simulink model "automatic_transmission_control"  (R2020b)
settings: Solver=ode5  StartTime=0.0  StopTime=30  FixedStep=0.001  RelTol=1e-3
PreLoadFcn:
  | initialization
values from neighbouring files (symbols this model uses):
  CONVERTER_DATA = [0 137.4652089938063 2.2319999999999998;0.1 137.06501915685197 2.075;0.2 135.86444964598905 1.975;0.30000000000000004 135.66435472751189 1.8459999999999999;0.4 137.56525645304487 1.72;0.5 140.36658531172509 1.564;0.60000000000000009 145.26891081441539 1.409;0.70000000000000007 152.87251771654735 1.254;0.8 162.97731109964374 1.0959999999999999;0.81 164.2779280697452 1.08;0.82000000000000006 166.178 ...(+346 chars)    [initialization.m]
  DOWN_TABLE = [0 5 20 35;0 5 20 35;0 5 25 40;0 5 30 50;0 30 50 80;0 30 50 80]    [initialization.m]
  DOWN_TH_BP = [0;5;40;50;90;100]    [initialization.m]
  EMAP = [-40 -44 -49 -53 -57 -61 -65 -70 -74 -78 -82;215 117 85 66 44 29 10 -2 -13 -22 -32;245 208 178 148 122 104 85 66 48 33 18;264 260 241 219 193 167 152 133 119 96 85;264 279 282 275 260 238 223 208 189 171 152;267 290 293 297 290 275 260 256 234 212 193;267 297 305 305 305 301 293 282 267 249 226;267 301 308 312 319 323 319 316 297 279 253;267 301 312 319 327 327 327 327 312 293 267;267 301 312 319  ...(+28 chars)    [initialization.m]
  Iei = 0.021991488283555904    (= 0.0219914882836)    [initialization.m]
  NE_VEC = [799.99999999999989 1200 1599.9999999999998 1999.9999999999998 2400 2800.0000000000005 3199.9999999999995 3599.9999999999995 3999.9999999999995 4400 4800]    [initialization.m]
  TH_VEC = [0;20;30;40;50;60;70;80;90;100]    [initialization.m]
  UP_TABLE = [10 30 50 1.0E+6;10 30 50 1.0E+6;15 30 50 1.0E+6;23 41 60 1.0E+6;40 70 100 1.0E+6;40 70 100 1.0E+6]    [initialization.m]
  UP_TH_BP = [0;25;35;50;90;100]    [initialization.m]
  VEHICLE_DATA = [3.23;40;0.02;1;12.094147857312473;0]    [initialization.m]
undefined symbols (not defined in the file or in its folder): sigbuilder_block
settings Model: Creator=Vrunda M Balgi  LastModifiedBy=Vrunda M Balgi

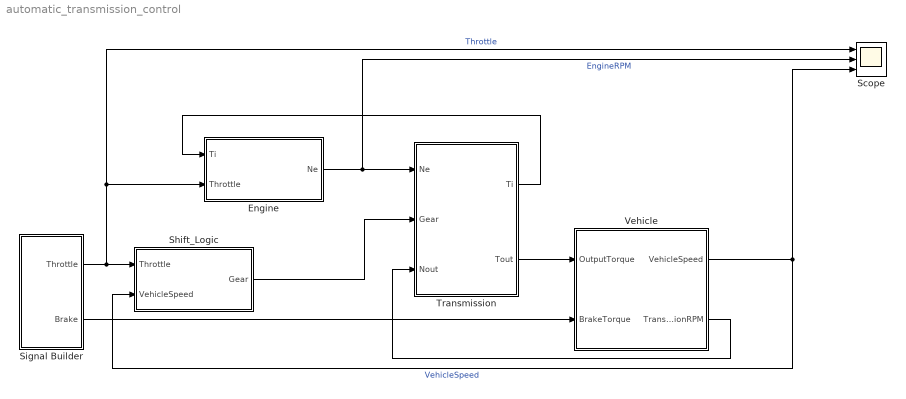
== system automatic_transmission_control ==
  Engine : Subsystem
  Scope : Scope  NumInputPorts=3
  Shift_Logic : Stateflow chart  TreatAsAtomicUnit=on
  Signal Builder : Subsystem  Tag=STV Subsys  LoadFcn=sigbuilder_block('load',[574.2 159.6 550.8 400.2 ]);  StartFcn=sigbuilder_block('start');  StopFcn=sigbuilder_block('stop');  ClipboardFcn=sigbuilder_block('clipboard');  mask(Sigbuilder block){tuvar=[0:10]}
      mask help: Simulink:masks:SigbuilderBlock_MD
      mask init:
      | if ~strcmp(get_param(bdroot(gcbh),'SimulationStatus'),'stopped') tuvar = sigbuilder_block('maskInit'); end
      settings: CopyFcn=sigbuilder_block('copy');  DeleteFcn=sigbuilder_block('delete');  ModelCloseFcn=sigbuilder_block('modelClose');  PreSaveFcn=sigbuilder_block('preSave');  PauseFcn=sigbuilder_block('pause');  ContinueFcn=sigbuilder_block('continue');  NameChangeFcn=sigbuilder_block('namechange');  OpenFcn=sigbuilder_block('open',[574.2 159.6 550.8 400.2 ]);  CloseFcn=sigbuilder_block('close');
      mask Display: plot(0, 0, 100, 100,[2, 2, 32, 32, 2], [68, 8, 8, 68, 68],[32, 2], [38, 38], [32, 19, 2],[53, 60, 44], [32, 17, 17, 2],[16, 16, 31, 31]);txt = getActiveGroup(gcbh);text(2, 100, txt,'verticalAlignment', 'top');
  Transmission : Subsystem
  Vehicle : Subsystem
  wires:
  Transmission/1(Ti) -> Engine/1(Ti)
  Signal Builder/1(Throttle) -> Scope/1, Engine/2(Throttle), Shift_Logic/1(Throttle)  "Throttle"
  Engine/1(Ne) -> Scope/2, Transmission/1(Ne)  "EngineRPM"
  Shift_Logic/1(Gear) -> Transmission/2(Gear)
  Vehicle/2(TransmissionRPM) -> Transmission/3(Nout)
  Transmission/2(Tout) -> Vehicle/1("OutputTorque ")
  Signal Builder/2(Brake) -> Vehicle/2(BrakeTorque)
  Vehicle/1(VehicleSpeed) -> Scope/3, Shift_Logic/2(VehicleSpeed)  "VehicleSpeed"

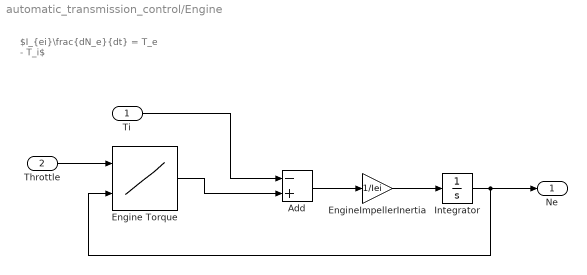
== system automatic_transmission_control/Engine ==
  note: $I_{ei}\frac{dN_e}{dt} = T_e - T_i$
  Ti : Inport  Unit=ft*lbf@torque
  Throttle : Inport  Port=2  Unit=%
  Add : Sum  Inputs=-+  InputSameDT=on  SaturateOnIntegerOverflow=on  OutDataTypeStr=Inherit: Same as first input
  Engine Torque : Lookup_n-D  BreakpointsForDimension1=TH_VEC  BreakpointsForDimension2=NE_VEC  BreakpointsForDimension3=[5, 7]  Table=EMAP  InputSameDT=on
      settings: InputPortMap=u0,u1
  EngineImpellerInertia : Gain  Gain=1/Iei  SaturateOnIntegerOverflow=on  OutDataTypeStr=Inherit: Same as input  ParamDataTypeStr=Inherit: Same as input
  Integrator : Integrator  InitialCondition=1000  LimitOutput=on  UpperSaturationLimit=6000  LowerSaturationLimit=600  ZeroCross=off
  Ne : Outport  Unit=rpm
  wires:
  Add/1 -> EngineImpellerInertia/1
  Throttle/1 -> Engine Torque/1
  Integrator/1 -> Ne/1, Engine Torque/2
  EngineImpellerInertia/1 -> Integrator/1
  Ti/1 -> Add/1
  Engine Torque/1 -> Add/2

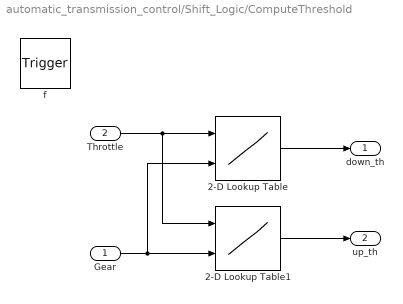
== system automatic_transmission_control/Shift_Logic/ComputeThreshold ==
  Gear : Inport  OutDataTypeStr=double  PortDimensions=1
  Throttle : Inport  Port=2  OutDataTypeStr=double  PortDimensions=1
  f : TriggerPort  TriggerType=function-call  VariantControl=(inherit)
      settings: CopyFcn=Stateflow.SLINSF.SimulinkMan.removeBlockPreDeleteFcn  PreDeleteFcn=Stateflow.SLINSF.SimulinkMan.unsafePredeleteFcn
  2-D Lookup Table : Lookup_n-D  BreakpointsForDimension1=UP_TH_BP  BreakpointsForDimension2=[1:4]  Table=UP_TABLE  OutDataTypeStr=double  LockScale=on
      settings: InputPortMap=u0,u1
  2-D Lookup Table1 : Lookup_n-D  BreakpointsForDimension1=DOWN_TH_BP  BreakpointsForDimension2=[1:4]  Table=DOWN_TABLE  OutDataTypeStr=double  InputSameDT=on
      settings: InputPortMap=u0,u1
  down_th : Outport
  up_th : Outport  Port=2
  wires:
  2-D Lookup Table/1 -> down_th/1
  Throttle/1 -> 2-D Lookup Table1/1, 2-D Lookup Table/1
  2-D Lookup Table1/1 -> up_th/1
  Gear/1 -> 2-D Lookup Table/2, 2-D Lookup Table1/2

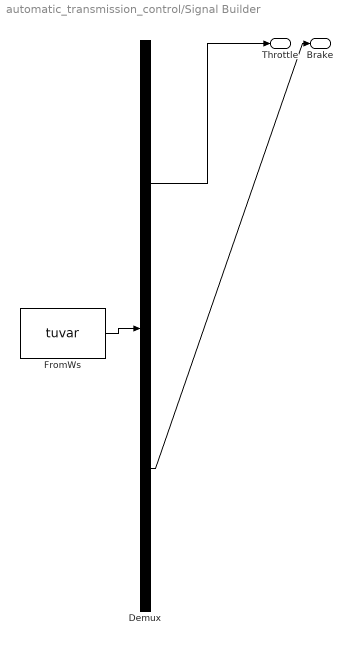
== system automatic_transmission_control/Signal Builder ==
  Demux : Demux  Tag=STV Demux  Outputs=2
      settings: DisplayOption=none
  FromWs : FromWorkspace  Tag=STV FromWs  VariableName=tuvar
      SigBuilderData=|
      | common.afterFinalStr = 'Extrapolate'
      | common.sampleTime = 0
      | dataSet(1).timeRange = [0 50]
      | dataSet(1).name = 'Passing Maneuver'
      | dataSet(2).timeRange = [0 50]
      | dataSet(2).name = 'Gradual Acceleration'
      | dataSet(3).timeRange = [0 50]
      | dataSet(3).name = 'Hard braking'
      | dataSet(4).timeRange = [0 50]
      | dataSet(4).name = 'Coasting'
      | sbobj.Groups(1).Name = 'Passing Maneuver'
      | sbobj.Groups(1).Signals(1).Name = 'Throttle'
      | sbobj.Groups(1).Signals(1).XData = [0 14.9 15 50]
      | sbobj.Groups(1).Signals(1).YData = [60 40 100 58.8235]
      | sbobj.Groups(1).Signals(2).Name = 'Brake'
      | sbobj.Groups(1).Signals(2).XData = [0 50]
      | sbobj.Groups(1).Signals(2).YData = [0 0]
      | sbobj.Groups(1).TimeRange = [0 50]
      | sbobj.Groups(2).Name = 'Gradual Acceleration'
      | sbobj.Groups(2).Signals(1).Name = 'Throttle'
      | sbobj.Groups(2).Signals(1).XData = [0 50]
      | sbobj.Groups(2).Signals(1).YData = [13.4 24]
      | sbobj.Groups(2).Signals(2).Name = 'Brake'
      | sbobj.Groups(2).Signals(2).XData = [0 50]
      | sbobj.Groups(2).Signals(2).YData = [0 0]
      | sbobj.Groups(2).TimeRange = [0 50]
      | sbobj.Groups(3).Name = 'Hard braking'
      | sbobj.Groups(3).Signals(1).Name = 'Throttle'
      | sbobj.Groups(3).Signals(1).XData = [0 5.1 5.1 50]
      | sbobj.Groups(3).Signals(1).YData = [50 50 1 1]
      | sbobj.Groups(3).Signals(2).Name = 'Brake'
      | sbobj.Groups(3).Signals(2).XData = [0 10 10 50]
      | sbobj.Groups(3).Signals(2).YData = [0 0 325 325]
      | sbobj.Groups(3).TimeRange = [0 50]
      | sbobj.Groups(4).Name = 'Coasting'
      | sbobj.Groups(4).Signals(1).Name = 'Throttle'
      | sbobj.Groups(4).Signals(1).XData = [0 4.8 4.8 50]
      | sbobj.Groups(4).Signals(1).YData = [80 80 1 1]
      | sbobj.Groups(4).Signals(2).Name = 'Brake'
      | sbobj.Groups(4).Signals(2).XData = [0 50]
      | sbobj.Groups(4).Signals(2).YData = [0 0]
      | sbobj.Groups(4).TimeRange = [0 50]
  Throttle : Outport  Tag=STV Outport
  Brake : Outport  Tag=STV Outport  Port=2
  wires:
  Demux/1 -> Throttle/1
  FromWs/1 -> Demux/1
  Demux/2 -> Brake/1

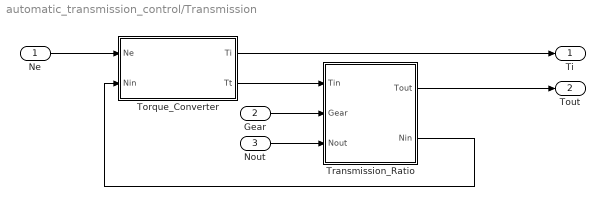
== system automatic_transmission_control/Transmission ==
  Ne : Inport  Unit=rpm
  Gear : Inport  Port=2  Unit=1
  Nout : Inport  Port=3  Unit=rpm
  Torque_Converter : Subsystem
  Transmission_Ratio : Subsystem
  Ti : Outport  Unit=ft*lbf@torque
  Tout : Outport  Port=2  Unit=ft*lbf@torque
  wires:
  Torque_Converter/1(Ti) -> Ti/1
  Ne/1 -> Torque_Converter/1(Ne)
  Nout/1 -> Transmission_Ratio/3(Nout)
  Transmission_Ratio/1(Tout) -> Tout/1
  Torque_Converter/2(Tt) -> Transmission_Ratio/1(Tin)
  Gear/1 -> Transmission_Ratio/2(Gear)
  Transmission_Ratio/2(Nin) -> Torque_Converter/2(Nin)

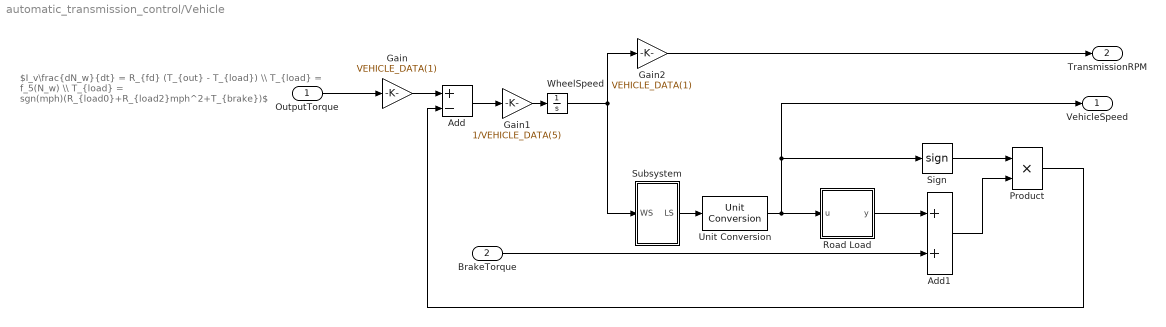
== system automatic_transmission_control/Vehicle ==
  note: $I_v\frac{dN_w}{dt} = R_{fd} (T_{out} - T_{load}) \\ T_{load} = f_5(N_w) \\ T_{load} = sgn(mph)(R_{load0}+R_{load2}mph^2+T_{brake})$
  "OutputTorque " : Inport  Unit=ft*lbf@torque
  BrakeTorque : Inport  Port=2
  Add : Sum  Inputs=+-  InputSameDT=on  SaturateOnIntegerOverflow=on  OutDataTypeStr=Inherit: Same as first input
  Add1 : Sum  InputSameDT=on  SaturateOnIntegerOverflow=on  OutDataTypeStr=Inherit: Same as first input
  Gain : Gain  Gain=VEHICLE_DATA(1)  SaturateOnIntegerOverflow=on  OutDataTypeStr=Inherit: Same as input  ParamDataTypeStr=Inherit: Same as input
  Gain1 : Gain  Gain=1/VEHICLE_DATA(5)  SaturateOnIntegerOverflow=on  OutDataTypeStr=Inherit: Same as input
  Gain2 : Gain  Gain=VEHICLE_DATA(1)  SaturateOnIntegerOverflow=on  OutDataTypeStr=Inherit: Same as input  ParamDataTypeStr=Inherit: Same as input
  Product : Product  InputSameDT=on  SaturateOnIntegerOverflow=on  OutDataTypeStr=Inherit: Same as first input
  Road Load : MATLAB Function  TreatAsAtomicUnit=on
  Sign : Signum  ZeroCross=off
  Subsystem : Subsystem
  Unit Conversion : UnitConversion
  WheelSpeed : Integrator  InitialCondition=(VEHICLE_DATA(6)/VEHICLE_DATA(4)*VEHICLE_DATA(1))/VEHICLE_DATA(1)  ZeroCross=off
  VehicleSpeed : Outport  Unit=mph
  TransmissionRPM : Outport  Port=2  Unit=rpm
  wires:
  Gain/1 -> Add/1
  Product/1 -> Add/2
  Unit Conversion/1 -> Road Load/1(u), VehicleSpeed/1, Sign/1
  Road Load/1(y) -> Add1/1
  "OutputTorque "/1 -> Gain/1
  Add1/1 -> Product/2
  Gain2/1 -> TransmissionRPM/1
  Add/1 -> Gain1/1
  Gain1/1 -> WheelSpeed/1
  Sign/1 -> Product/1
  Subsystem/1(LS) -> Unit Conversion/1
  BrakeTorque/1 -> Add1/2
  WheelSpeed/1 -> Subsystem/1(WS), Gain2/1

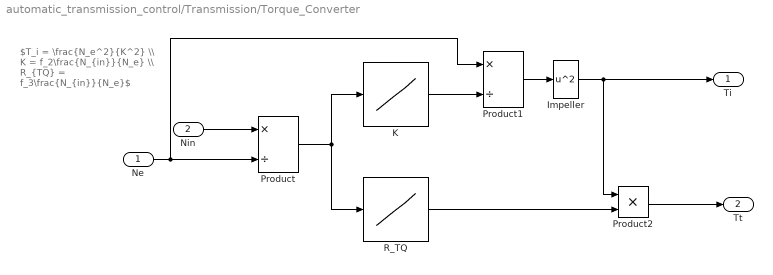
== system automatic_transmission_control/Transmission/Torque_Converter ==
  note: $T_i = \frac{N_e^2}{K^2} \\ K = f_2\frac{N_{in}}{N_e} \\ R_{TQ} = f_3\frac{N_{in}}{N_e}$
  Ne : Inport
  Nin : Inport  Port=2
  Impeller : Fcn  Expr=u^2
  K : Lookup_n-D  NumberOfTableDimensions=1  BreakpointsForDimension1=CONVERTER_DATA(:,1)  Table=CONVERTER_DATA(:,2)  SaturateOnIntegerOverflow=on  InputSameDT=on
  Product : Product  Inputs=*/  InputSameDT=on  SaturateOnIntegerOverflow=on  OutDataTypeStr=Inherit: Same as first input
  Product1 : Product  Inputs=*/  InputSameDT=on  SaturateOnIntegerOverflow=on  OutDataTypeStr=Inherit: Same as first input
  Product2 : Product  InputSameDT=on  SaturateOnIntegerOverflow=on  OutDataTypeStr=Inherit: Same as first input
  R_TQ : Lookup_n-D  NumberOfTableDimensions=1  BreakpointsForDimension1=CONVERTER_DATA(:,1)  Table=CONVERTER_DATA(:,3)  SaturateOnIntegerOverflow=on  InputSameDT=on
  Ti : Outport
  Tt : Outport  Port=2
  wires:
  Product/1 -> R_TQ/1, K/1
  Product2/1 -> Tt/1
  K/1 -> Product1/2
  R_TQ/1 -> Product2/2
  Product1/1 -> Impeller/1
  Impeller/1 -> Ti/1, Product2/1
  Ne/1 -> Product1/1, Product/2
  Nin/1 -> Product/1

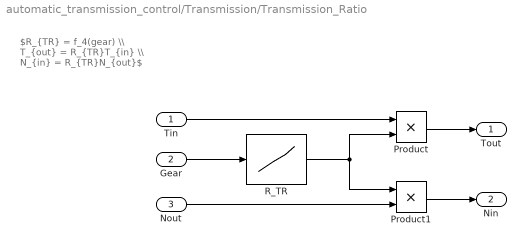
== system automatic_transmission_control/Transmission/Transmission_Ratio ==
  note: $R_{TR} = f_4(gear) \\ T_{out} = R_{TR}T_{in} \\ N_{in} = R_{TR}N_{out}$
  Tin : Inport  Unit=ft*lbf@torque
  Gear : Inport  Port=2  Unit=1
  Nout : Inport  Port=3  Unit=rpm
  Product : Product  InputSameDT=on  SaturateOnIntegerOverflow=on  OutDataTypeStr=Inherit: Same as first input
  Product1 : Product  InputSameDT=on  SaturateOnIntegerOverflow=on  OutDataTypeStr=Inherit: Same as first input
  R_TR : Lookup_n-D  NumberOfTableDimensions=1  BreakpointsForDimension1=[1 2 3 4]  Table=[2.393 1.450 1.000 0.677]  OutDataTypeStr=double  SaturateOnIntegerOverflow=on  InputSameDT=on  LockScale=on
  Tout : Outport  Unit=ft*lbf@torque
  Nin : Outport  Port=2  Unit=rpm
  wires:
  Tin/1 -> Product/1
  Product/1 -> Tout/1
  Nout/1 -> Product1/2
  Product1/1 -> Nin/1
  R_TR/1 -> Product/2, Product1/1
  Gear/1 -> R_TR/1

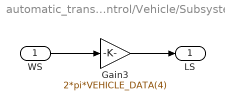
== system automatic_transmission_control/Vehicle/Subsystem ==
  WS : Inport  Unit=rpm
  Gain3 : Gain  Gain=2*pi*VEHICLE_DATA(4)  SaturateOnIntegerOverflow=on  OutDataTypeStr=Inherit: Same as input  ParamDataTypeStr=Inherit: Same as input
  LS : Outport  Unit=ft/min
  wires:
  WS/1 -> Gain3/1
  Gain3/1 -> LS/1

== matlab function automatic_transmission_control/Vehicle/Road Load ==
  data: u input; y output
function y = fcn(u)
rload0 = 40;
rload2 = 0.0200;

y = rload0+(rload2*u*u);
end

== stateflow chart automatic_transmission_control/Shift_Logic ==
  state GearState [parallel]
    settings: executionOrder=1
    state first
      entry:
      Gear = 1;
    state second
      entry:
      Gear = 2;
    state third
      entry:
      Gear = 3;
    state fourth
      entry:
      Gear = 4;
    (default) -> first
    first -> second : UP
    second -> third [order 1] : UP
    third -> fourth [order 1] : UP
    fourth -> third : DOWN
    third -> second [order 2] : DOWN
    second -> first [order 2] : DOWN
  state SelectionAction [parallel]
    during:
    [down_th,up_th] = ComputeThreshold(Gear,Throttle);
    settings: executionOrder=2
    state steady_state
    state down_shift
    state up_shift
    (default) -> steady_state
    steady_state -> up_shift [order 1] : [VehicleSpeed>up_th]
    steady_state -> down_shift [order 2] : [VehicleSpeed<down_th]
    down_shift -> steady_state [order 1] : after(TWAIT,tick)
        | [VehicleSpeed<=down_th]
        | {GearState.DOWN}
    down_shift -> steady_state [order 2] : [VehicleSpeed>down_th]
    up_shift -> steady_state [order 1] : after(TWAIT,tick)
        | [VehicleSpeed>=up_th]
        | {GearState.UP}
    up_shift -> steady_state [order 2] : [VehicleSpeed<up_th]
  state [down_th,up_th] = ComputeThreshold(Gear,Throttle) [function]
  data: Gear function_input double size=1; Throttle function_input double size=1; down_th function_output; up_th function_output; Gear output; Throttle input; VehicleSpeed input; down_th local; up_th local; TWAIT parameter
  events: DOWN local FUNCTION_CALL_EVENT; UP local FUNCTION_CALL_EVENT
